simulink model "PL2_Velocidad_Controlador_Optimal"  (R2021b)
settings: Solver=VariableStepAuto  StartTime=0.0  StopTime=1  RelTol=1e-3
values from neighbouring files (symbols this model uses):
  B = (0.01*TN)/WN    (= 1.7806207167e-07)    [PL2_Velocidad_optimal_m.m]
  J = 4.28*(10^(-7))    (= 4.28e-07)    [PL2_Velocidad_optimal_m.m]
  KB = 1/((557)*(pi)/30)    (= 0.0171441590404)    [PL2_Velocidad_optimal_m.m]
  KT = 17.2*10^(-3)    (= 0.0172)    [PL2_Velocidad_optimal_m.m]
  LA = 0.2*10^(-3)    (= 0.0002)    [PL2_Velocidad_optimal_m.m]
  RA = 4.05    [PL2_Velocidad_optimal_m.m]
  TORC = 6*10^-3    (= 0.006)    [PL2_Velocidad_optimal_m.m]
settings Model: Creator=яблоня  LastModifiedBy=Elvis

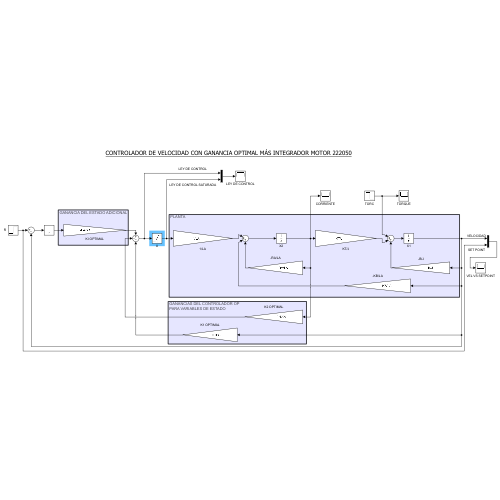
[thumbnail: Simulink's stored preview of the top-level diagram]
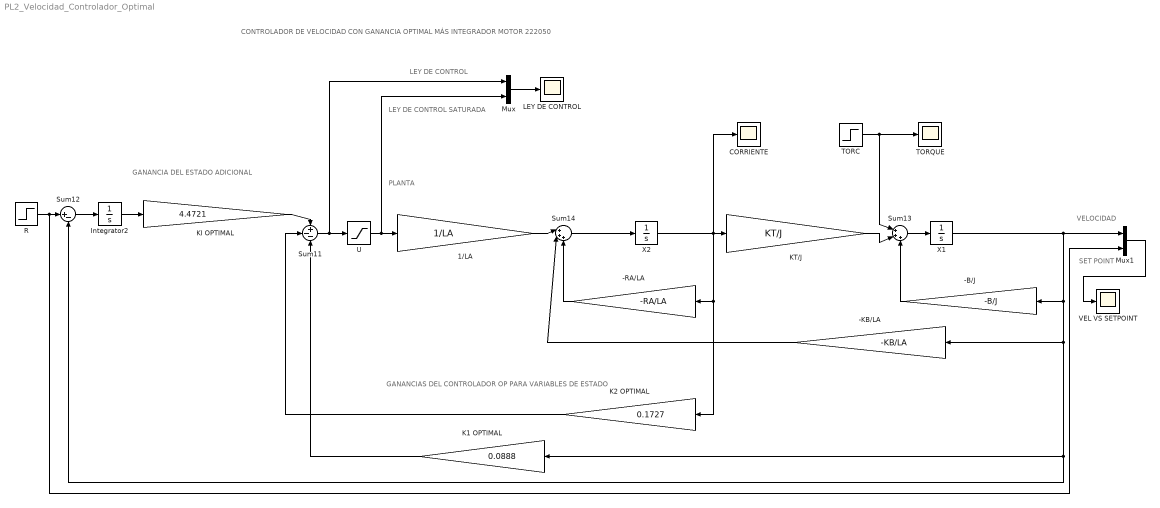
== system PL2_Velocidad_Controlador_Optimal ==
  note: CONTROLADOR DE VELOCIDAD CON GANANCIA OPTIMAL MÁS INTEGRADOR MOTOR 222050
  note: GANANCIA DEL ESTADO ADICIONAL
  note: GANANCIAS DEL CONTROLADOR OP
      | PARA VARIABLES DE ESTADO
  note: SET POINT
  note: VELOCIDAD
  note: LEY DE CONTROL
  note: LEY DE CONTROL SATURADA
  note: PLANTA
  -B/J : Gain  Gain=-B/J
  -KB/LA : Gain  Gain=-KB/LA
  -RA/LA : Gain  Gain=-RA/LA
  1/LA : Gain  Gain=1/LA
  CORRIENTE : Scope
  Integrator2 : Integrator
  K1 OPTIMAL : Gain  Gain=0.0888
  K2 OPTIMAL : Gain  Gain=0.1727
  KI OPTIMAL : Gain  Gain=4.4721
  KT/J : Gain  Gain=KT/J
  LEY DE CONTROL : Scope
  Mux : Mux  Inputs=2
  Mux1 : Mux  Inputs=2
  R : Step  Time=0  Before=500  After=500  SampleTime=0
  Sum11 : Sum  Inputs=+--
  Sum12 : Sum  Inputs=|+-
  Sum13 : Sum  Inputs=|+++
  Sum14 : Sum  Inputs=|+++
  TORC : Step  Time=0  After=-TORC/J  SampleTime=0
  TORQUE : Scope
  U : Saturate  UpperLimit=15  LowerLimit=-15
  VEL VS SETPOINT : Scope
  X1 : Integrator
  X2 : Integrator
  wires:
  KI OPTIMAL/1 -> Sum11/1
  U/1 -> Mux/2, 1/LA/1
  X2/1 -> CORRIENTE/1, -RA/LA/1, K2 OPTIMAL/1, KT/J/1
  Sum12/1 -> Integrator2/1
  1/LA/1 -> Sum14/1
  Integrator2/1 -> KI OPTIMAL/1
  -KB/LA/1 -> Sum14/2
  TORC/1 -> TORQUE/1, Sum13/1
  K1 OPTIMAL/1 -> Sum11/3
  Sum13/1 -> X1/1
  -B/J/1 -> Sum13/3
  Sum14/1 -> X2/1
  KT/J/1 -> Sum13/2
  X1/1 -> Mux1/1, -B/J/1, -KB/LA/1, Sum12/2, K1 OPTIMAL/1
  Sum11/1 -> Mux/1, U/1
  K2 OPTIMAL/1 -> Sum11/2
  -RA/LA/1 -> Sum14/3
  R/1 -> Mux1/2, Sum12/1
  Mux/1 -> LEY DE CONTROL/1
  Mux1/1 -> VEL VS SETPOINT/1
